simulink model "Exercitiul4"  (R2016a)
settings: Solver=VariableStepDiscrete  StartTime=0.0  StopTime=960  RelTol=1e-3
undefined symbols (not defined in the file): m, n
settings Model: Creator=Cristina  LastModifiedBy=Cristina

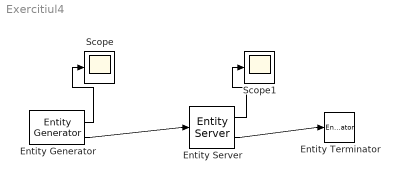
== system Exercitiul4 ==
  Entity Generator : EntityGenerator  OutputPortMessageModes=n,m  TimeSource=MATLAB action  IntergenerationTimeAction=dt = 12 + 12 * rand;  NumberEntitiesDeparted=on  EntityType=Structured  EntityTypeName=Entity
      settings: OutputPortMap=o0,o3
  Entity Server : EntityServer  InputPortMessageModes=m  OutputPortMessageModes=n,m  Capacity=2  ServiceTimeSource=MATLAB action  ServiceTimeAction=dt = 28 + 8 * rand;  NumberEntitiesDeparted=on
      settings: OutputPortMap=o0,o9
  Entity Terminator : EntityTerminator  InputPortMessageModes=m
  Scope : Scope
  Scope1 : Scope
  wires:
  Entity Server/2 -> Entity Terminator/1
  Entity Generator/2 -> Entity Server/1
  Entity Generator/1 -> Scope/1
  Entity Server/1 -> Scope1/1
